simulink model "pedal_post_logic_and_sensor"  (R2024b)
settings: Solver=FixedStepDiscrete  StartTime=0.0  StopTime=1  RelTol=1e-3
libraries: simulink x1
settings Model: Creator=Ahmed  LastModifiedBy=Ahmed

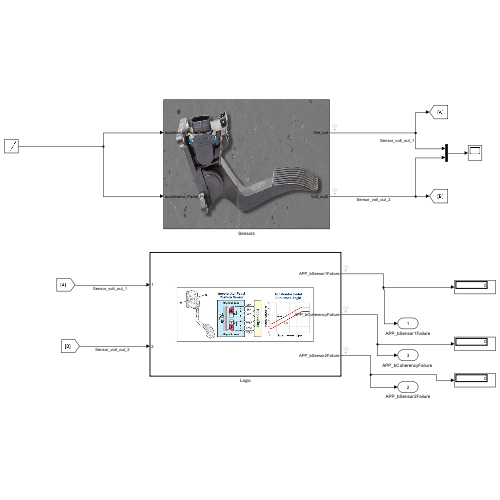
[thumbnail: Simulink's stored preview of the top-level diagram]
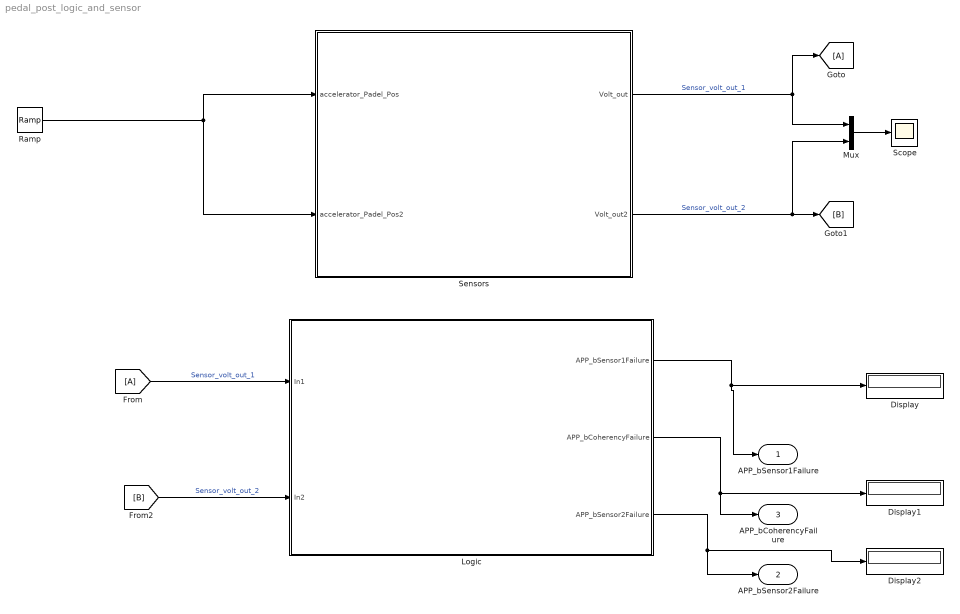
== system pedal_post_logic_and_sensor ==
  Display : Display
  Display1 : Display
  Display2 : Display
  From : From
  Goto : Goto
  Logic : Subsystem  TreatAsAtomicUnit=on
      mask Display: image('FAST-5-APS-Pedal-Angle.jpg', [0,0,0,0,75,75]);
  Mux : Mux  Inputs=2
  Ramp : simulink/Sources/Ramp  slope=1  start=0  InitialOutput=0
  Scope : Scope
  Sensors : Subsystem
      mask Display: image('accelerator-pedal-position-sensor-e1720492592554.jpg');
  APP_bSensor1Failure : Outport
  APP_bSensor2Failure : Outport  Port=2
  "APP_bCoherencyFailure " : Outport  Port=3
  wires:
  Ramp/1 -> Sensors/2(accelerator_Padel_Pos2), Sensors/1(accelerator_Padel_Pos)
  Sensors/1(Volt_out) -> Mux/1, Goto/1  "Sensor_volt_out_1"
  Sensors/2(Volt_out2) -> Mux/2, [B]  "Sensor_volt_out_2"
  From/1 -> Logic/1(In1)  "Sensor_volt_out_1"
  [B] -> Logic/2(In2)  "Sensor_volt_out_2"
  Logic/1(APP_bSensor1Failure) -> APP_bSensor1Failure/1, Display/1
  Logic/2(APP_bCoherencyFailure) -> "APP_bCoherencyFailure "/1, Display1/1
  Logic/3(APP_bSensor2Failure) -> APP_bSensor2Failure/1, Display2/1
  Mux/1 -> Scope/1

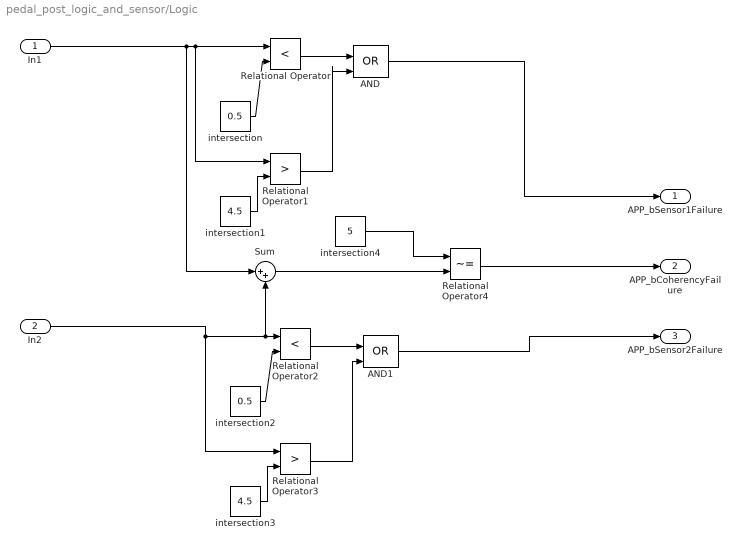
== system pedal_post_logic_and_sensor/Logic ==
  In1 : Inport
  In2 : Inport  Port=2
  AND : Logic  Operator=OR  IconShape=distinctive  AllPortsSameDT=off  OutDataTypeStr=boolean
  AND1 : Logic  Operator=OR  IconShape=distinctive  AllPortsSameDT=off  OutDataTypeStr=boolean
  Relational Operator : RelationalOperator  Operator=<  OutDataTypeStr=boolean  RndMeth=Simplest  InputSameDT=off
  Relational Operator1 : RelationalOperator  Operator=>  OutDataTypeStr=boolean  RndMeth=Simplest  InputSameDT=off
  Relational Operator2 : RelationalOperator  Operator=<  OutDataTypeStr=boolean  RndMeth=Simplest  InputSameDT=off
  Relational Operator3 : RelationalOperator  Operator=>  OutDataTypeStr=boolean  RndMeth=Simplest  InputSameDT=off
  Relational Operator4 : RelationalOperator  Operator=~=  OutDataTypeStr=boolean  RndMeth=Simplest  InputSameDT=off
  Sum : Sum  Inputs=|++
  intersection : Constant  Value=0.5
  intersection1 : Constant  Value=4.5
  intersection2 : Constant  Value=0.5
  intersection3 : Constant  Value=4.5
  intersection4 : Constant  Value=5
  APP_bSensor1Failure : Outport
  APP_bCoherencyFailure : Outport  Port=2
  APP_bSensor2Failure : Outport  Port=3
  wires:
  intersection4/1 -> Relational Operator4/1
  Relational Operator/1 -> AND/1
  Relational Operator4/1 -> APP_bCoherencyFailure/1
  intersection/1 -> Relational Operator/2
  Sum/1 -> Relational Operator4/2
  intersection2/1 -> Relational Operator2/2
  intersection1/1 -> Relational Operator1/2
  Relational Operator1/1 -> AND/2
  In2/1 -> Sum/2, Relational Operator2/1, Relational Operator3/1
  AND1/1 -> APP_bSensor2Failure/1
  In1/1 -> Sum/1, Relational Operator/1, Relational Operator1/1
  Relational Operator3/1 -> AND1/2
  Relational Operator2/1 -> AND1/1
  intersection3/1 -> Relational Operator3/2
  AND/1 -> APP_bSensor1Failure/1

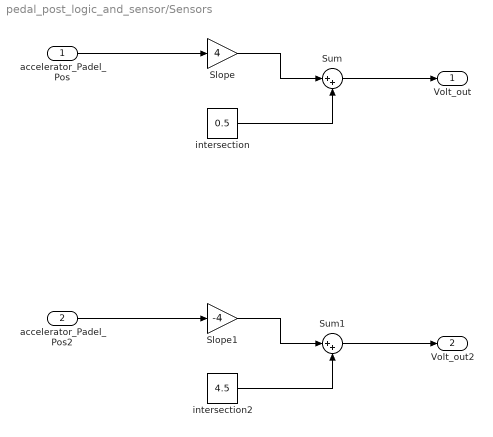
== system pedal_post_logic_and_sensor/Sensors ==
  accelerator_Padel_Pos : Inport
  accelerator_Padel_Pos2 : Inport  Port=2
  Slope : Gain  Gain=4
  Slope1 : Gain  Gain=-4
  Sum : Sum  Inputs=|++
  Sum1 : Sum  Inputs=|++
  intersection : Constant  Value=0.5
  "intersection2 " : Constant  Value=4.5
  Volt_out : Outport
  Volt_out2 : Outport  Port=2
  wires:
  Sum1/1 -> Volt_out2/1
  intersection/1 -> Sum/2
  Sum/1 -> Volt_out/1
  Slope1/1 -> Sum1/1
  accelerator_Padel_Pos/1 -> Slope/1
  "intersection2 "/1 -> Sum1/2
  accelerator_Padel_Pos2/1 -> Slope1/1
  Slope/1 -> Sum/1
